simulink model "tasks"  (R2018a)
settings: Solver=VariableStepAuto  StartTime=0.0  StopTime=10.0  RelTol=1e-3
undefined symbols (not defined in the file or in its folder): sigbuilder_block
settings Model: EnablePacing=on  Creator=U500304  LastModifiedBy=U500304

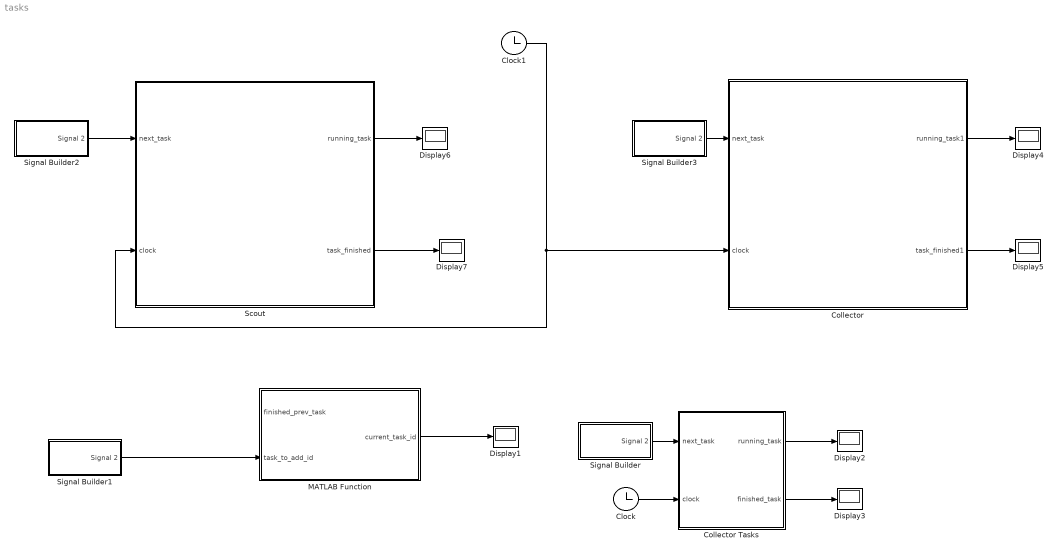
== system tasks ==
  Clock : Clock
  Clock1 : Clock
  "Collector " : Subsystem
  Collector Tasks : Stateflow chart  TreatAsAtomicUnit=on
  Display{1..7} (7 alike) : Display
  MATLAB Function : MATLAB Function  TreatAsAtomicUnit=on
  Scout : Subsystem
  Signal Builder : Subsystem  Tag=STV Subsys  LoadFcn=sigbuilder_block('load');  StartFcn=sigbuilder_block('start');  StopFcn=sigbuilder_block('stop');  ClipboardFcn=sigbuilder_block('clipboard');  mask(Sigbuilder block){tuvar=[0:10]}
      mask help: Simulink:masks:SigbuilderBlock_MD
      mask init:
      | if ~strcmp(get_param(bdroot(gcbh),'SimulationStatus'),'stopped') tuvar = sigbuilder_block('maskInit'); end
      settings: CopyFcn=sigbuilder_block('copy');  DeleteFcn=sigbuilder_block('delete');  ModelCloseFcn=sigbuilder_block('modelClose');  PreSaveFcn=sigbuilder_block('preSave');  PauseFcn=sigbuilder_block('pause');  ContinueFcn=sigbuilder_block('continue');  NameChangeFcn=sigbuilder_block('namechange');  OpenFcn=sigbuilder_block('open',[327 53.4 550.8 361.2 ]);  CloseFcn=sigbuilder_block('close');
      mask Display: plot(0, 0, 100, 100,[2, 2, 32, 32, 2], [68, 8, 8, 68, 68],[32, 2], [38, 38], [32, 19, 2],[53, 60, 44], [32, 17, 17, 2],[16, 16, 31, 31]);txt = getActiveGroup(gcbh);text(2, 100, txt,'verticalAlignment', 'top');
  Signal Builder1 : Subsystem  Tag=STV Subsys  LoadFcn=sigbuilder_block('load');  StartFcn=sigbuilder_block('start');  StopFcn=sigbuilder_block('stop');  ClipboardFcn=sigbuilder_block('clipboard');  mask(Sigbuilder block){tuvar=[0:10]}
      mask help: Simulink:masks:SigbuilderBlock_MD
      mask init:
      | if ~strcmp(get_param(bdroot(gcbh),'SimulationStatus'),'stopped') tuvar = sigbuilder_block('maskInit'); end
      settings: CopyFcn=sigbuilder_block('copy');  DeleteFcn=sigbuilder_block('delete');  ModelCloseFcn=sigbuilder_block('modelClose');  PreSaveFcn=sigbuilder_block('preSave');  PauseFcn=sigbuilder_block('pause');  ContinueFcn=sigbuilder_block('continue');  NameChangeFcn=sigbuilder_block('namechange');  OpenFcn=sigbuilder_block('open',[327 53.4 550.8 361.2 ]);  CloseFcn=sigbuilder_block('close');
      mask Display: plot(0, 0, 100, 100,[2, 2, 32, 32, 2], [68, 8, 8, 68, 68],[32, 2], [38, 38], [32, 19, 2],[53, 60, 44], [32, 17, 17, 2],[16, 16, 31, 31]);txt = getActiveGroup(gcbh);text(2, 100, txt,'verticalAlignment', 'top');
  Signal Builder2 : Subsystem  Tag=STV Subsys  LoadFcn=sigbuilder_block('load');  StartFcn=sigbuilder_block('start');  StopFcn=sigbuilder_block('stop');  ClipboardFcn=sigbuilder_block('clipboard');  mask(Sigbuilder block){tuvar=[0:10]}
      mask help: Simulink:masks:SigbuilderBlock_MD
      mask init:
      | if ~strcmp(get_param(bdroot(gcbh),'SimulationStatus'),'stopped') tuvar = sigbuilder_block('maskInit'); end
      settings: CopyFcn=sigbuilder_block('copy');  DeleteFcn=sigbuilder_block('delete');  ModelCloseFcn=sigbuilder_block('modelClose');  PreSaveFcn=sigbuilder_block('preSave');  PauseFcn=sigbuilder_block('pause');  ContinueFcn=sigbuilder_block('continue');  NameChangeFcn=sigbuilder_block('namechange');  OpenFcn=sigbuilder_block('open',[327 53.4 550.8 361.2 ]);  CloseFcn=sigbuilder_block('close');
      mask Display: plot(0, 0, 100, 100,[2, 2, 32, 32, 2], [68, 8, 8, 68, 68],[32, 2], [38, 38], [32, 19, 2],[53, 60, 44], [32, 17, 17, 2],[16, 16, 31, 31]);txt = getActiveGroup(gcbh);text(2, 100, txt,'verticalAlignment', 'top');
  Signal Builder3 : Subsystem  Tag=STV Subsys  LoadFcn=sigbuilder_block('load');  StartFcn=sigbuilder_block('start');  StopFcn=sigbuilder_block('stop');  ClipboardFcn=sigbuilder_block('clipboard');  mask(Sigbuilder block){tuvar=[0:10]}
      mask help: Simulink:masks:SigbuilderBlock_MD
      mask init:
      | if ~strcmp(get_param(bdroot(gcbh),'SimulationStatus'),'stopped') tuvar = sigbuilder_block('maskInit'); end
      settings: CopyFcn=sigbuilder_block('copy');  DeleteFcn=sigbuilder_block('delete');  ModelCloseFcn=sigbuilder_block('modelClose');  PreSaveFcn=sigbuilder_block('preSave');  PauseFcn=sigbuilder_block('pause');  ContinueFcn=sigbuilder_block('continue');  NameChangeFcn=sigbuilder_block('namechange');  OpenFcn=sigbuilder_block('open',[327 53.4 550.8 361.2 ]);  CloseFcn=sigbuilder_block('close');
      mask Display: plot(0, 0, 100, 100,[2, 2, 32, 32, 2], [68, 8, 8, 68, 68],[32, 2], [38, 38], [32, 19, 2],[53, 60, 44], [32, 17, 17, 2],[16, 16, 31, 31]);txt = getActiveGroup(gcbh);text(2, 100, txt,'verticalAlignment', 'top');
  wires:
  Collector Tasks/1(running_task) -> Display2/1
  Clock/1 -> Collector Tasks/2(clock)
  Signal Builder/1(Signal 2) -> Collector Tasks/1(next_task)
  Signal Builder1/1(Signal 2) -> MATLAB Function/2(task_to_add_id)
  MATLAB Function/1(current_task_id) -> Display1/1
  Collector Tasks/2(finished_task) -> Display3/1
  "Collector "/1(running_task1) -> Display4/1
  "Collector "/2(task_finished1) -> Display5/1
  Scout/1(running_task) -> Display6/1
  Scout/2(task_finished) -> Display7/1
  Clock1/1 -> Scout/2("clock "), "Collector "/2("clock ")
  Signal Builder2/1(Signal 2) -> Scout/1(next_task)
  Signal Builder3/1(Signal 2) -> "Collector "/1(next_task)

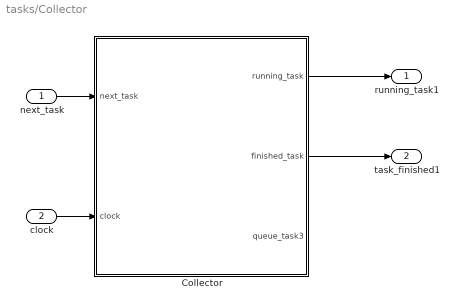
== system tasks/Collector  ==
  next_task : Inport
  "clock " : Inport  Port=2
  Collector : Stateflow chart  TreatAsAtomicUnit=on
  running_task1 : Outport
  task_finished1 : Outport  Port=2
  wires:
  next_task/1 -> Collector/1(next_task)
  "clock "/1 -> Collector/2(clock)
  Collector/2(" finished_task") -> task_finished1/1
  Collector/1(running_task) -> running_task1/1

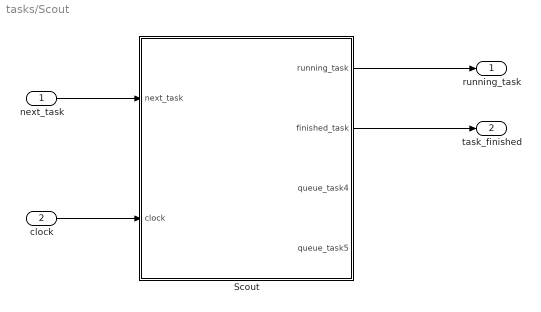
== system tasks/Scout ==
  next_task : Inport
  "clock " : Inport  Port=2
  Scout : Stateflow chart  TreatAsAtomicUnit=on
  running_task : Outport
  task_finished : Outport  Port=2
  wires:
  next_task/1 -> Scout/1(next_task)
  Scout/1(running_task) -> running_task/1
  "clock "/1 -> Scout/2(clock)
  Scout/2(" finished_task") -> task_finished/1

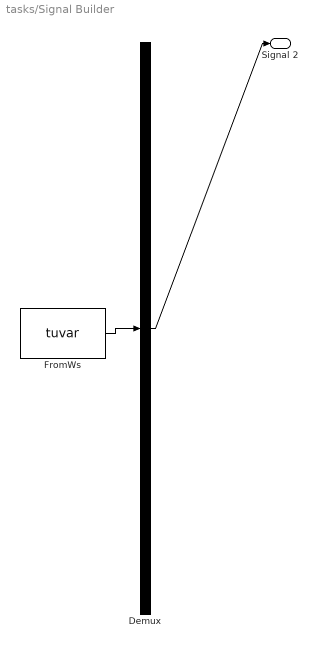
== system tasks/Signal Builder ==
  Demux : Demux  Tag=STV Demux  Outputs=1
  FromWs : FromWorkspace  Tag=STV FromWs  VariableName=tuvar  SampleTime=0
      SigBuilderData=|
      | common.afterFinalStr = 'Extrapolate'
      | common.sampleTime = 0
      | dataSet.timeRange = [0 10]
      | dataSet.name = 'Group 1'
      | sbobj.Groups.Name = 'Group 1'
      | sbobj.Groups.Signals.Name = 'Signal 2'
      | sbobj.Groups.Signals.XData = [0 0.5 0.5 1 1 1.5 2 2.5 3 3.5 4 4.5 5 5.5 6 6 6.5 6.5 7 7.5 8 8.5 9 9.5 10]
      | sbobj.Groups.Signals.YData = [0.01 0.01 1 1 0 0 0 0 0 0 0 0 0 0 0 2 2 0 0 0 0 0 0 0 0]
  Signal 2 : Outport  Tag=STV Outport
  wires:
  FromWs/1 -> Demux/1
  Demux/1 -> Signal 2/1

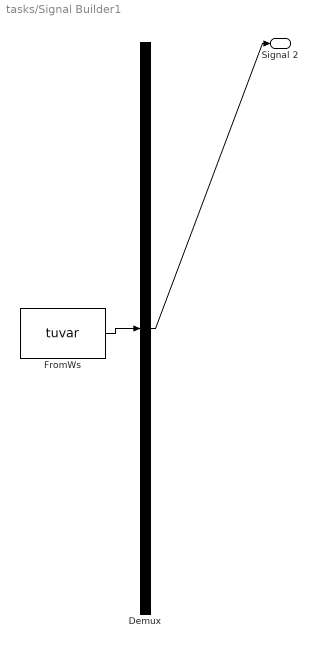
== system tasks/Signal Builder1 ==
  Demux : Demux  Tag=STV Demux  Outputs=1
  FromWs : FromWorkspace  Tag=STV FromWs  VariableName=tuvar  SampleTime=0
      SigBuilderData=|
      | common.afterFinalStr = 'Extrapolate'
      | common.sampleTime = 0
      | dataSet.timeRange = [0 10]
      | dataSet.name = 'Group 1'
      | sbobj.Groups.Name = 'Group 1'
      | sbobj.Groups.Signals.Name = 'Signal 2'
      | sbobj.Groups.Signals.XData = [0 0.5 0.5 2 2 2.5 3 3 4.5 4.5 5 5.5 6 6 8 8 8.5 9 9.5 10]
      | sbobj.Groups.Signals.YData = [0.01 0.01 1 1 0 0 0 3 3 0 0 0 0 2 2 0 0 0 0 0]
  Signal 2 : Outport  Tag=STV Outport
  wires:
  Demux/1 -> Signal 2/1
  FromWs/1 -> Demux/1

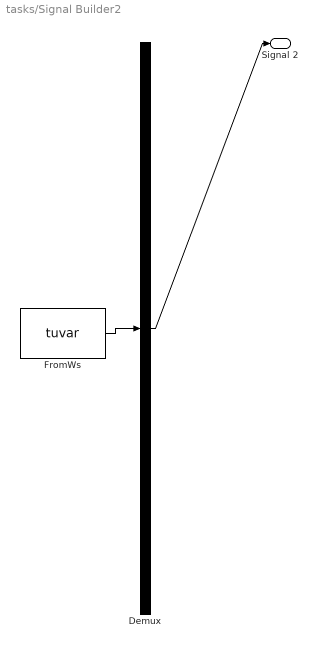
== system tasks/Signal Builder2 ==
  Demux : Demux  Tag=STV Demux  Outputs=1
  FromWs : FromWorkspace  Tag=STV FromWs  VariableName=tuvar  SampleTime=0
      SigBuilderData=|
      | common.afterFinalStr = 'Extrapolate'
      | common.sampleTime = 0
      | dataSet.timeRange = [0 10]
      | dataSet.name = 'Group 1'
      | sbobj.Groups.Name = 'Group 1'
      | sbobj.Groups.Signals.Name = 'Signal 2'
      | sbobj.Groups.Signals.XData = [0 0.5 0.5 1 1 1.5 2 2.5 3 3.5 4 4.5 5 5.5 6 6 6.5 6.5 7 7.5 8 8.5 9 9.5 10]
      | sbobj.Groups.Signals.YData = [0.01 0.01 1 1 0 0 0 0 0 0 0 0 0 0 0 2 2 0 0 0 0 0 0 0 0]
  Signal 2 : Outport  Tag=STV Outport
  wires:
  Demux/1 -> Signal 2/1
  FromWs/1 -> Demux/1

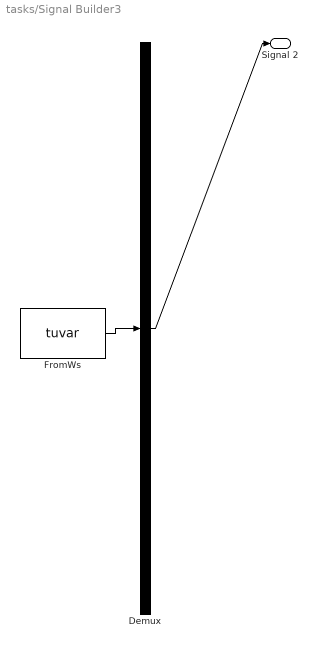
== system tasks/Signal Builder3 ==
  Demux : Demux  Tag=STV Demux  Outputs=1
  FromWs : FromWorkspace  Tag=STV FromWs  VariableName=tuvar  SampleTime=0
      SigBuilderData=|
      | common.afterFinalStr = 'Extrapolate'
      | common.sampleTime = 0
      | dataSet.timeRange = [0 10]
      | dataSet.name = 'Group 1'
      | sbobj.Groups.Name = 'Group 1'
      | sbobj.Groups.Signals.Name = 'Signal 2'
      | sbobj.Groups.Signals.XData = [0 0.5 0.5 2 2 2.5 3 3 4.5 4.5 5 5.5 6 6 8 8 8.5 9 9.5 10]
      | sbobj.Groups.Signals.YData = [0.01 0.01 1 1 0 0 0 3 3 0 0 0 0 2 2 0 0 0 0 0]
  Signal 2 : Outport  Tag=STV Outport
  wires:
  FromWs/1 -> Demux/1
  Demux/1 -> Signal 2/1

== matlab function tasks/MATLAB Function ==
  data: finished_prev_task input; current_task_id output; task_to_add_id input
function current_task_id = schedule_tasklist(finished_prev_task, task_to_add_id)
current_task_id = 0;

coder.updateBuildInfo('addSourceFiles','taskList.c');
coder.cinclude('taskList.h');

%current_task = struct();
%coder.cstructname(current_task,'task','extern','HeaderFile','taskList.h');
%new_task = struct();
%coder.cstructname(new_task,'task','extern','HeaderFile','taskList.h');

%tasks = struct();
%coder.cstructname(tasks,'task_list','extern','HeaderFile','taskList.h');
new_task = 0;
coder.ceval('initialize_task_list_matlab');
%new_task = coder.ceval('create_task_matlab', 004);
coder.ceval('accept_task_matlab', 004);
current_task = 0;
current_task = coder.ceval('pop_task_matlab');
current_task_id = current_task;

while 0
    if (task_to_add_id > 0 && task_to_add_id ~= current_task_id)
        new_task = coder.ceval('create_task', task_to_add_id);
        coder.ceval('accept_task', new_task, coder.ref(tasks));
    end
    if finished_prev_task
        current_task = coder.ceval('pop_task', coder.ref(tasks));
        current_task_id = coder.ceval('get_task_id', coder.ref(current_task));
    end
    
    if task_to_add_id > 9
        break
    end
end   
    
end

== stateflow chart tasks/Scout/Scout ==
  settings: updateMethod=CONTINUOUS
  note: Placeholder for real task data
  state Schedule
  state Orientation_and_Drive
    en:
    running_task = 0;
    timer = clock;
  state Generate_New_Goal
    en:
    running_task = 1;
    timer = clock;
    cost = 12;
  state Communicate_Own_Position
    en:
    running_task = 2;
    timer = clock;
    cost = 5;
  state Receive_Photo_Sensor_Readings
    en:
    running_task = 3;
    timer = clock;
    cost = 10;
  state Handle_High_Readings
    en:
    running_task = 4;
    timer = clock;
    cost = 4;
  state Communicate_Harvest_Coordinates
    en:
    running_task = 5;
    timer = clock;
    cost = 5;
  state Receive_Referee_Communication
    en:
    running_task = 6;
    timer = clock;
    cost = 7;
  (default) -> Schedule : {next_task; clock;}
  Schedule -> Orientation_and_Drive [order 3] : [next_task == 0]
  Orientation_and_Drive -> Schedule : [next_task ~= 0]
  Schedule -> Generate_New_Goal [order 2] : [next_task == 1]
  Generate_New_Goal -> Schedule : [clock - timer > cost]
  Schedule -> Communicate_Own_Position [order 1] : [next_task == 2]
  Communicate_Own_Position -> Schedule : [clock - timer > cost]
  Schedule -> Receive_Photo_Sensor_Readings [order 4] : [next_task == 3]
  Receive_Photo_Sensor_Readings -> Schedule : [clock - timer > cost]
  Schedule -> Handle_High_Readings [order 5] : [next_task == 4]
  Handle_High_Readings -> Schedule : [clock - timer > cost]
  Schedule -> Communicate_Harvest_Coordinates [order 6] : [next_task == 5]
  Communicate_Harvest_Coordinates -> Schedule : [clock - timer > cost]
  Schedule -> Receive_Referee_Communication [order 7] : [next_task == 6]
  Receive_Referee_Communication -> Schedule : [clock - timer > cost]
  data: next_task input; cost local; timer local; running_task output; clock input; finished_task output boolean; queue_task4 output boolean; queue_task5 output boolean
  data timer settings: updateMethod=SF_CONTINUOUS_TIME_DATA

== stateflow chart tasks/Collector Tasks ==
  settings: updateMethod=CONTINUOUS
  note: Placeholder for real task data
  state Schedule
  state Idle1
    en:
    running_task = 0;
    timer = clock;
  state Task1
    en:
    running_task = 1;
    timer = clock;
    cost = 3;
  state Task2
    en:
    running_task = 2;
    timer = clock;
    cost = 5;
  state Task3
    en:
    running_task = 3;
    timer = clock;
    cost = 5;
  state Task4
    en:
    running_task = 4;
    timer = clock;
    cost = 5;
  state Task5
    en:
    running_task = 5;
    timer = clock;
    cost = 5;
  state Task6
    en:
    running_task = 6;
    timer = clock;
    cost = 5;
  state Task7
    en:
    running_task = 7;
    timer = clock;
    cost = 5;
  (default) -> Schedule : {next_task; clock;}
  Schedule -> Idle1 [order 3] : [next_task == 0]
  Idle1 -> Schedule : [next_task ~= 0]
  Schedule -> Task1 [order 2] : [next_task == 1]
  Task1 -> Schedule : [clock - timer > cost]
  Schedule -> Task2 [order 1] : [next_task == 2]
  Task2 -> Schedule : [clock - timer > cost]
  Schedule -> Task3 [order 4] : [next_task == 3]
  Task3 -> Schedule : [clock - timer > cost]
  Schedule -> Task4 [order 5] : [next_task == 4]
  Task4 -> Schedule : [clock - timer > cost]
  Schedule -> Task5 [order 6] : [next_task == 5]
  Task5 -> Schedule : [clock - timer > cost]
  Schedule -> Task6 [order 7] : [next_task == 6]
  Task6 -> Schedule : [clock - timer > cost]
  Schedule -> Task7 [order 8] : [next_task == 7]
  Task7 -> Schedule : [clock - timer > cost]
  data: next_task input; cost local; timer local; running_task output; clock input; finished_task output boolean
  data timer settings: updateMethod=SF_CONTINUOUS_TIME_DATA

== stateflow chart tasks/Collector /Collector ==
  settings: updateMethod=CONTINUOUS
  note: Placeholder for real task data
  state Schedule
  state Orientation_and_Drive
    en:
    running_task = 0;
    timer = clock;
  state Generate_New_Goal
    en:
    running_task = 1;
    timer = clock;
    cost = 12;
  state Receive_Proximity_Sensor_Readings
    en:
    running_task = 2;
    timer = clock;
    cost = 8;
  state Handle_High_Readings
    en:
    running_task = 3;
    timer = clock;
    cost = 10;
  state Receive_Harvest_Coordinates
    en:
    running_task = 4;
    timer = clock;
    cost = 5;
  state Receive_Referee_Communication
    en:
    running_task = 5;
    timer = clock;
    cost = 5;
  (default) -> Schedule : {next_task; clock;}
  Schedule -> Orientation_and_Drive [order 2] : [next_task == 0]
  Orientation_and_Drive -> Schedule : [next_task ~= 0]
  Schedule -> Generate_New_Goal [order 1] : [next_task == 1]
  Generate_New_Goal -> Schedule : [clock - timer > cost]
  Schedule -> Receive_Proximity_Sensor_Readings [order 3] : [next_task == 2]
  Receive_Proximity_Sensor_Readings -> Schedule : [clock - timer > cost]
  Schedule -> Handle_High_Readings [order 4] : [next_task == 3]
  Handle_High_Readings -> Schedule : [clock - timer > cost]
  Schedule -> Receive_Harvest_Coordinates [order 5] : [next_task == 4]
  Receive_Harvest_Coordinates -> Schedule : [clock - timer > cost]
  Schedule -> Receive_Referee_Communication [order 6] : [next_task == 5]
  Receive_Referee_Communication -> Schedule : [clock - timer > cost]
  data: next_task input; cost local; timer local; running_task output; clock input; finished_task output boolean; queue_task3 output boolean
  data timer settings: updateMethod=SF_CONTINUOUS_TIME_DATA
